simulink model "mobile_robot_diffdrive"  (R2025b)
settings: Solver=ode1  StartTime=0.0  StopTime=inf  FixedStep=0.1  RelTol=1e-3
model workspace (MAT data in the model file):
  example_omega_ts = timeseries
  example_omega_ts.Name = 'example_omega_ts'
  example_omega_ts.DataInfo = tsdata.datametadata
  example_omega_ts.DataInfo.Interpolation = tsdata.interpolation
  example_omega_ts.DataInfo.Interpolation.Fhandle : function handle (value not decoded)
  example_omega_ts.DataInfo.Interpolation.Name = 'linear'
  example_omega_ts.TimeInfo = tsdata.timemetadata
  example_omega_ts.TimeInfo.Length = 3001
  example_omega_ts.TimeInfo.DuplicateTimes = 0
  example_omega_ts.TimeInfo.Time_ = [0 0.02 0.04 0.06 0.08 0.1 0.12 0.14 0.16 0.18 0.2 0.22 ... (3001 elements, 3001x1)]
  example_omega_ts.TimeInfo.Initialized = 1
  example_omega_ts.QualityInfo = tsdata.qualmetadata
  example_omega_ts.Data_ = [0 0 0 0 0 0 0 0 0 0 0 0 ... (3001 elements, 3001x1)]
  example_v_ts = timeseries
  example_v_ts.Name = 'example_v_ts'
  example_v_ts.DataInfo = tsdata.datametadata
  example_v_ts.DataInfo.Interpolation = tsdata.interpolation
  example_v_ts.DataInfo.Interpolation.Fhandle : function handle (value not decoded)
  example_v_ts.DataInfo.Interpolation.Name = 'linear'
  example_v_ts.TimeInfo = tsdata.timemetadata
  example_v_ts.TimeInfo.Length = 3001
  example_v_ts.TimeInfo.DuplicateTimes = 0
  example_v_ts.TimeInfo.Time_ = [0 0.02 0.04 0.06 0.08 0.1 0.12 0.14 0.16 0.18 0.2 0.22 ... (3001 elements, 3001x1)]
  example_v_ts.TimeInfo.Initialized = 1
  example_v_ts.QualityInfo = tsdata.qualmetadata
  example_v_ts.Data_ = [0.25 0.25 0.25 0.25 0.25 0.25 0.25 0.25 0.25 0.25 0.25 0.25 ... (3001 elements, 3001x1)]
libraries: SignalEditorBlockLib x1
settings Model: SimulationMode=accelerator  Creator=Bender  LastModifiedBy=Bender

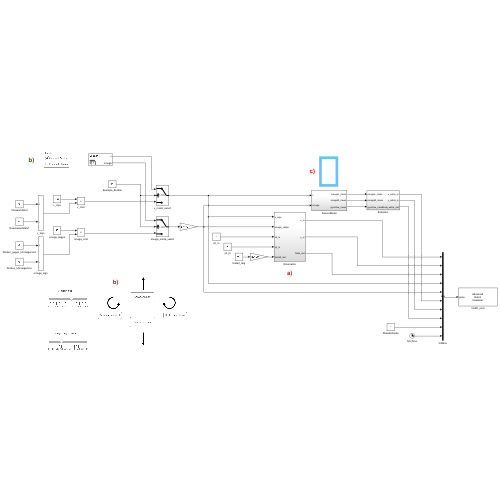
[thumbnail: Simulink's stored preview of the top-level diagram]
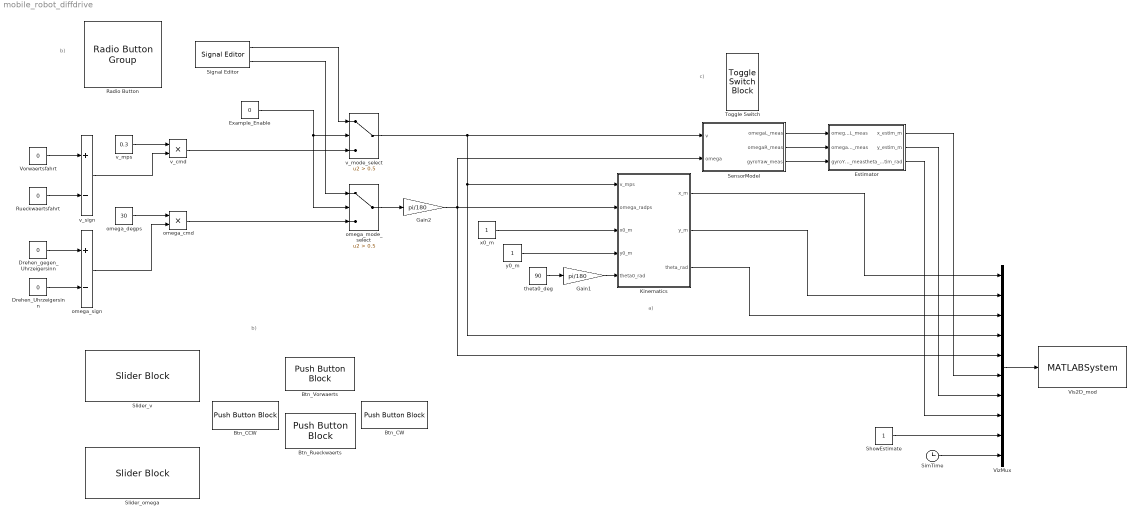
== system mobile_robot_diffdrive ==
  note: a)
  note: b)
  note: b)
  note: c)
  Btn_CCW : PushButtonBlock  ButtonText=Drehen - gegen Uhrzeigersinn  IconOnColor=[0.0, 0.39215686274509803, 0.0]  IconOffColor=[0.0, 1.0, 0.0]  OffValue=0.000000
  Btn_CW : PushButtonBlock  ButtonText=Drehen - im Uhrzeigersinn  IconOnColor=[0.0, 0.39215686274509803, 0.0]  IconOffColor=[0.0, 1.0, 0.0]  OffValue=0.000000
  Btn_Rueckwaerts : PushButtonBlock  ButtonText=Rueckwaertsfahrt  IconOnColor=[0.0, 0.39215686274509803, 0.0]  IconOffColor=[0.0, 1.0, 0.0]  OffValue=0.000000
  Btn_Vorwaerts : PushButtonBlock  ButtonText=Vorwaertsfahrt  IconOnColor=[0.0, 0.39215686274509803, 0.0]  IconOffColor=[0.0, 1.0, 0.0]  OffValue=0.000000
  Drehen_Uhrzeigersinn : Constant  Value=0
  Drehen_gegen_Uhrzeigersinn : Constant  Value=0
  Estimator : Subsystem
  Example_Enable : Constant  Value=0
  Gain1 : Gain  Gain=pi/180
  Gain2 : Gain  Gain=pi/180
  Kinematics : Subsystem
  Radio Button : RadioButtonGroup  LabelPosition=Hide  SelectedLabel=Manual Control  ButtonGroupName=Inputs
  Rueckwaertsfahrt : Constant  Value=0
  SensorModel : Subsystem
  ShowEstimate : Constant
  Signal Editor : SignalEditorBlockLib/Signal Editor  FileName=exampleSig.mat  ActiveScenario=Scenario  ActiveSignal=v  IsBus=off  OutputBusObjectStr=Bus: BusObject  SampleTime=0  ZeroCross=off  OutputAfterFinalValue=Setting to zero  Unit=inherit  PreserveSignalName=on  ApplySigPropsToAllScenarios=on  ApplySigPropsToAllSignals=off  SignalPropertySource=Dialog parameters
  SimTime : Clock
  Slider_omega : SliderBlock  ScaleMax=90
  Slider_v : SliderBlock  ScaleMax=0.5
  Toggle Switch : ToggleSwitchBlock
  Vis2D_mod : MATLABSystem  System=Visualizer2D_advanced  robotRadius=0.1  showPath=on  showTimeTrajectories=on  hasWaypoints=off  hasLidar=off  sensorOffset=[ 0, 0 ]  scanAngles=[ -pi / 4, 0, pi / 4 ]  hasObjDetector=off  objDetectorOffset=[ 0, 0 ]  objDetectorAngle=0  objDetectorFOV=pi / 4  objDetectorMaxRange=5  objectColors=[ 1, 0, 0; 0, 1, 0; 0, 0, 1 ]  objectMarkers=s
      mask Type: Visualizer2D_advanced
  VizMux : Mux  Inputs=10
  Vorwaertsfahrt : Constant  Value=0
  omega_cmd : Product
  omega_degps : Constant  Value=30
  omega_mode_select : Switch  Criteria=u2 > Threshold  Threshold=0.5  SaturateOnIntegerOverflow=off  InputSameDT=off
  omega_sign : Sum  Inputs=+-
  theta0_deg : Constant  Value=90
  v_cmd : Product
  v_mode_select : Switch  Criteria=u2 > Threshold  Threshold=0.5  SaturateOnIntegerOverflow=off  InputSameDT=off
  v_mps : Constant  Value=0.3
  v_sign : Sum  Inputs=+-
  x0_m : Constant
  y0_m : Constant
  wires:
  Vorwaertsfahrt/1 -> v_sign/1
  omega_sign/1 -> omega_cmd/2
  v_sign/1 -> v_cmd/2
  Rueckwaertsfahrt/1 -> v_sign/2
  omega_degps/1 -> omega_cmd/1
  Estimator/3(theta_estim_rad) -> VizMux/8
  Drehen_gegen_Uhrzeigersinn/1 -> omega_sign/1
  v_mps/1 -> v_cmd/1
  Drehen_Uhrzeigersinn/1 -> omega_sign/2
  Example_Enable/1 -> omega_mode_select/2, v_mode_select/2
  SimTime/1 -> VizMux/10
  v_cmd/1 -> v_mode_select/3
  Estimator/2(y_estim_m) -> VizMux/7
  omega_cmd/1 -> omega_mode_select/3
  v_mode_select/1 -> VizMux/4, Kinematics/1(v_mps), SensorModel/1(v)
  Kinematics/1(x_m) -> VizMux/1
  Kinematics/2(y_m) -> VizMux/2
  Kinematics/3(theta_rad) -> VizMux/3
  Estimator/1(x_estim_m) -> VizMux/6
  ShowEstimate/1 -> VizMux/9
  SensorModel/1(omegaL_meas) -> Estimator/1(omegaL_meas)
  SensorModel/2(omegaR_meas) -> Estimator/2(omegaR_meas)
  SensorModel/3(gyroYaw_meas) -> Estimator/3(gyroYaw_meas)
  Signal Editor/1 -> v_mode_select/1
  Signal Editor/2 -> omega_mode_select/1
  x0_m/1 -> Kinematics/3(x0_m)
  y0_m/1 -> Kinematics/4(y0_m)
  theta0_deg/1 -> Gain1/1
  omega_mode_select/1 -> Gain2/1
  Gain1/1 -> Kinematics/5(theta0_rad)
  Gain2/1 -> SensorModel/2(omega), Kinematics/2(omega_radps), VizMux/5
  VizMux/1 -> Vis2D_mod/1

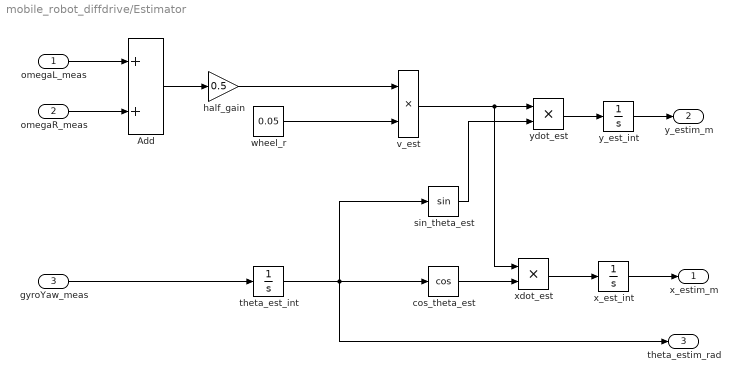
== system mobile_robot_diffdrive/Estimator ==
  omegaL_meas : Inport
  omegaR_meas : Inport  Port=2
  gyroYaw_meas : Inport  Port=3
  Add : Sum
  cos_theta_est : Trigonometry  Operator=cos
  half_gain : Gain  Gain=0.5
  sin_theta_est : Trigonometry
  theta_est_int : Integrator  InitialCondition=pi/2
  v_est : Product
  wheel_r : Constant  Value=0.05
  x_est_int : Integrator  InitialCondition=1
  xdot_est : Product
  y_est_int : Integrator  InitialCondition=1
  ydot_est : Product
  x_estim_m : Outport
  y_estim_m : Outport  Port=2
  theta_estim_rad : Outport  Port=3
  wires:
  omegaL_meas/1 -> Add/1
  omegaR_meas/1 -> Add/2
  Add/1 -> half_gain/1
  half_gain/1 -> v_est/1
  wheel_r/1 -> v_est/2
  gyroYaw_meas/1 -> theta_est_int/1
  theta_est_int/1 -> cos_theta_est/1, sin_theta_est/1, theta_estim_rad/1
  v_est/1 -> xdot_est/1, ydot_est/1
  cos_theta_est/1 -> xdot_est/2
  sin_theta_est/1 -> ydot_est/2
  xdot_est/1 -> x_est_int/1
  ydot_est/1 -> y_est_int/1
  x_est_int/1 -> x_estim_m/1
  y_est_int/1 -> y_estim_m/1

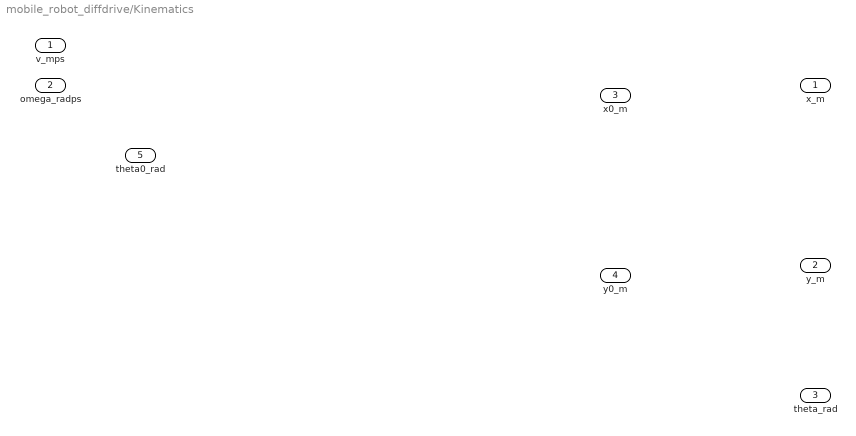
== system mobile_robot_diffdrive/Kinematics ==
  v_mps : Inport
  omega_radps : Inport  Port=2
  x0_m : Inport  Port=3
  y0_m : Inport  Port=4
  theta0_rad : Inport  Port=5
  x_m : Outport
  y_m : Outport  Port=2
  theta_rad : Outport  Port=3

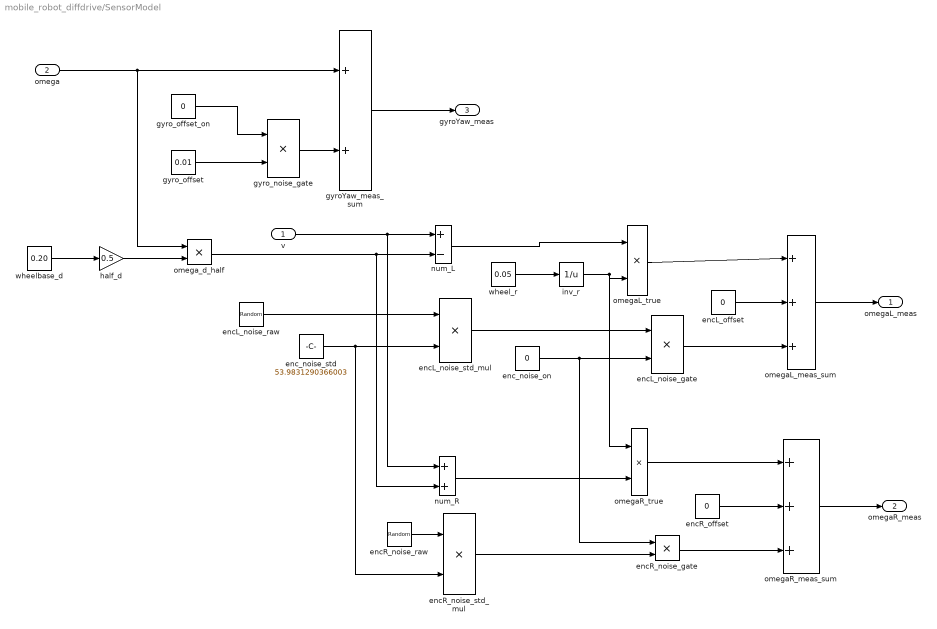
== system mobile_robot_diffdrive/SensorModel ==
  v : Inport
  omega : Inport  Port=2
  encL_noise_gate : Product
  encL_noise_raw : RandomNumber  SampleTime=0.1
  encL_noise_std_mul : Product
  encL_offset : Constant  Value=0
  encR_noise_gate : Product
  encR_noise_raw : RandomNumber  SampleTime=0.1
  encR_noise_std_mul : Product
  encR_offset : Constant  Value=0
  enc_noise_on : Constant  Value=0
  enc_noise_std : Constant  Value=53.9831290366003
  gyroYaw_meas_sum : Sum
  gyro_noise_gate : Product
  gyro_offset : Constant  Value=0.01
  gyro_offset_on : Constant  Value=0
  half_d : Gain  Gain=0.5
  inv_r : Math  Operator=reciprocal
  num_L : Sum  Inputs=+-
  num_R : Sum
  omegaL_meas_sum : Sum  Inputs=+++
  omegaL_true : Product
  omegaR_meas_sum : Sum  Inputs=+++
  omegaR_true : Product
  omega_d_half : Product
  wheel_r : Constant  Value=0.05
  wheelbase_d : Constant  Value=0.20
  omegaL_meas : Outport
  omegaR_meas : Outport  Port=2
  gyroYaw_meas : Outport  Port=3
  wires:
  encR_noise_std_mul/1 -> encR_noise_gate/2
  gyro_offset/1 -> gyro_noise_gate/2
  omegaL_meas_sum/1 -> omegaL_meas/1
  encR_noise_gate/1 -> omegaR_meas_sum/3
  encL_noise_raw/1 -> encL_noise_std_mul/1
  num_L/1 -> omegaL_true/1
  wheelbase_d/1 -> half_d/1
  omega/1 -> omega_d_half/1, gyroYaw_meas_sum/1
  inv_r/1 -> omegaR_true/1, omegaL_true/2
  half_d/1 -> omega_d_half/2
  gyroYaw_meas_sum/1 -> gyroYaw_meas/1
  v/1 -> num_R/1, num_L/1
  omega_d_half/1 -> num_L/2, num_R/2
  wheel_r/1 -> inv_r/1
  omegaL_true/1 -> omegaL_meas_sum/1
  enc_noise_std/1 -> encL_noise_std_mul/2, encR_noise_std_mul/2
  encR_noise_raw/1 -> encR_noise_std_mul/1
  encL_noise_std_mul/1 -> encL_noise_gate/1
  num_R/1 -> omegaR_true/2
  enc_noise_on/1 -> encL_noise_gate/2, encR_noise_gate/1
  encL_offset/1 -> omegaL_meas_sum/2
  encL_noise_gate/1 -> omegaL_meas_sum/3
  omegaR_true/1 -> omegaR_meas_sum/1
  encR_offset/1 -> omegaR_meas_sum/2
  omegaR_meas_sum/1 -> omegaR_meas/1
  gyro_noise_gate/1 -> gyroYaw_meas_sum/2
  gyro_offset_on/1 -> gyro_noise_gate/1
